simulink model "ParallelControl"  (R2015b)
settings: Solver=ode45  StartTime=0.0  StopTime=10  FixedStep=.002  RelTol=1e-3
settings Model: ExtModeTrigDuration=10000  Creator=smascaro  LastModifiedBy=Justin
settings SolverCC: PositivePriorityOrder=on
settings DataIOCC: LimitDataPoints=off  SaveFormat=Array  SignalLoggingSaveFormat=ModelDataLogs  SaveOutput=off  SaveTime=off
settings OptimizationCC: ExpressionDepthLimit=2147483647  InitFltsAndDblsToZero=on
settings DebuggingCC: SaveWithParameterizedLinksMsg=none  UnderspecifiedInitializationDetection=Classic  MergeDetectMultiDrivingBlocksExec=none  SignalResolutionControl=TryResolveAllWithWarning  SolverPrmCheckMsg=warning  MultiTaskDSMMsg=warning  MultiTaskCondExecSysMsg=none  FcnCallInpInsideContextMsg=UseLocalSettings  StateNameClashWarn=warning
settings HardwareCC: ProdBitPerPointer=32  ProdLargestAtomicFloat=None  ProdIntDivRoundTo=Undefined  ProdEndianess=Unspecified  ProdWordSize=32  ProdHWDeviceType=32-bit Generic  TargetBitPerPointer=64  TargetLongLongMode=on  TargetIntDivRoundTo=Zero  TargetEndianess=LittleEndian  TargetWordSize=64  TargetHWDeviceType=MATLAB Host
settings SFSimCC: SimParseCustomCode=off
settings RTWCC: SystemTargetFile=quarc_windows.tlc  TemplateMakefile=quarc_default_tmf  Description=QUARC Win32 Target
settings STFCustomTargetCC: TargetPreCompLibLocation=C:\PROGRA~3\QUARC\lib\2015b\windows\release  ConcurrentExecutionCompliant=off  SystemTargetFile=quarc_windows.tlc
settings GRTTargetCC: TargetPreCompLibLocation=C:\PROGRA~3\QUARC\lib\2015b\windows\release  ParMdlRefBuildCompliant=off  CompOptLevelCompliant=off  ConcurrentExecutionCompliant=off  GeneratePreprocessorConditionals=Disable all  CombineOutputUpdateFcns=off  MatFileLogging=off  GRTInterface=on  UseToolchainInfoCompliant=off  ExtMode=on  ExtModeMexFile=quarc_comm
settings ConfigComp: CovModelRefEnable=Off

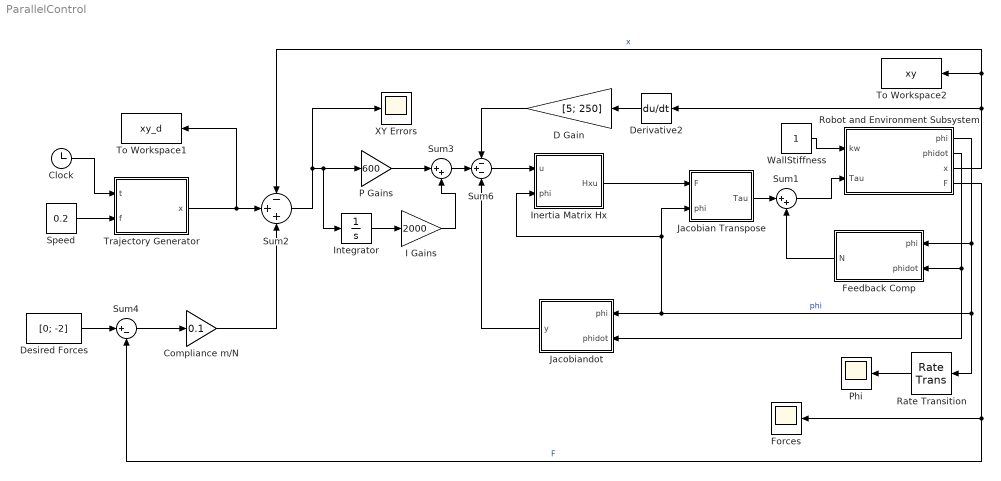
== system ParallelControl ==
  Clock : Clock
  "Compliance m/N " : Gain  Gain=0.1
  D Gain : Gain  Gain=[5; 250]
  Derivative2 : Derivative
  Desired Forces : Constant  Value=[0; -2]
  Feedback Comp : MATLAB Function  TreatAsAtomicUnit=on
  Forces : Scope
  I Gains : Gain  Gain=2000
  Inertia Matrix Hx : MATLAB Function  TreatAsAtomicUnit=on
  Integrator : Integrator
  Jacobian Transpose : MATLAB Function  TreatAsAtomicUnit=on
  Jacobiandot : MATLAB Function  TreatAsAtomicUnit=on
  P Gains : Gain  Gain=600
  Phi : Scope
      settings: AttributesFormatString=SampleTime =%<SampleTime>
  Rate Transition : RateTransition  OutPortSampleTimeOpt=Inherit  OutPortSampleTimeMultiple=10  OutPortSampleTime=0.05
  Robot and Environment Subsystem : Subsystem
  Speed : Constant  Value=0.2
      settings: AttributesFormatString=(circles/sec)
  Sum1 : Sum  Inputs=|++
  Sum2 : Sum  Inputs=-++
  Sum3 : Sum  Inputs=|++
  Sum4 : Sum  Inputs=|+-
  Sum6 : Sum  Inputs=-+-
  To Workspace1 : ToWorkspace  VariableName=xy_d  SampleTime=-1
  To Workspace2 : ToWorkspace  VariableName=xy  SampleTime=-1
  Trajectory Generator : MATLAB Function  TreatAsAtomicUnit=on
  WallStiffness : Constant
      settings: AttributesFormatString=(N/mm)
  XY Errors : Scope
  wires:
  Robot and Environment Subsystem/1(phi) -> Feedback Comp/1(phi), Jacobian Transpose/2(phi), Inertia Matrix Hx/2(phi), Jacobiandot/1(phi), Rate Transition/1  "phi"
  Robot and Environment Subsystem/3(x) -> To Workspace2/1, Sum2/1, Derivative2/1  "x"
  Clock/1 -> Trajectory Generator/1(t)
  Speed/1 -> Trajectory Generator/2(f)
  Rate Transition/1 -> Phi/1
  Robot and Environment Subsystem/4(F) -> Forces/1, Sum4/2  "F"
  Jacobian Transpose/1(Tau) -> Sum1/1
  Robot and Environment Subsystem/2(phidot) -> Jacobiandot/2(phidot), Feedback Comp/2(phidot)
  Feedback Comp/1(N) -> Sum1/2
  Sum1/1 -> Robot and Environment Subsystem/2(Tau)
  WallStiffness/1 -> Robot and Environment Subsystem/1(kw)
  Trajectory Generator/1(x) -> To Workspace1/1, Sum2/2
  Derivative2/1 -> D Gain/1
  Desired Forces/1 -> Sum4/1
  Sum4/1 -> "Compliance m/N "/1
  D Gain/1 -> Sum6/1
  Sum6/1 -> Inertia Matrix Hx/1(u)
  Inertia Matrix Hx/1(Hxu) -> Jacobian Transpose/1(F)
  "Compliance m/N "/1 -> Sum2/3
  Jacobiandot/1(y) -> Sum6/3
  Sum2/1 -> Integrator/1, P Gains/1, XY Errors/1
  Integrator/1 -> I Gains/1
  P Gains/1 -> Sum3/1
  Sum3/1 -> Sum6/2
  I Gains/1 -> Sum3/2

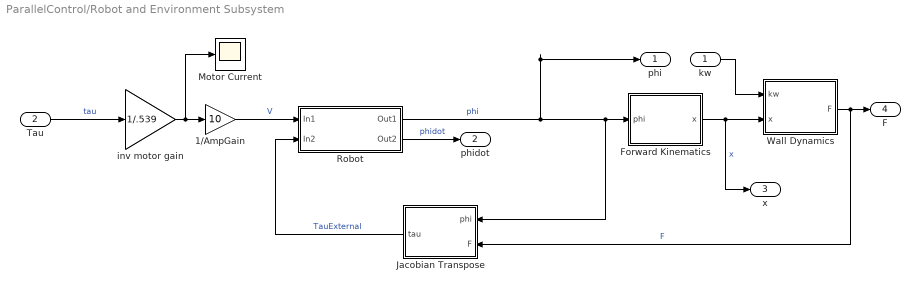
== system ParallelControl/Robot and Environment Subsystem ==
  kw : Inport
  Tau : Inport  Port=2
  1/AmpGain : Gain  Gain=10
  Forward Kinematics : MATLAB Function  TreatAsAtomicUnit=on
  Jacobian Transpose : MATLAB Function  TreatAsAtomicUnit=on
  Motor Current : Scope
  Robot : Subsystem
      mask Display: disp('Manipulator')
  Wall Dynamics : MATLAB Function  TreatAsAtomicUnit=on
  inv motor gain : Gain  Gain=1/.539
  phi : Outport
  phidot : Outport  Port=2
  x : Outport  Port=3
  F : Outport  Port=4
  wires:
  Robot/1(Out1) -> phi/1, Jacobian Transpose/1(phi), Forward Kinematics/1(phi)  "phi"
  Forward Kinematics/1(x) -> x/1, Wall Dynamics/2(x)  "x"
  Wall Dynamics/1(F) -> Jacobian Transpose/2(F), F/1  "F"
  inv motor gain/1 -> 1/AmpGain/1, Motor Current/1
  1/AmpGain/1 -> Robot/1(In1)  "V"
  kw/1 -> Wall Dynamics/1(kw)
  Robot/2(Out2) -> phidot/1  "phidot"
  Tau/1 -> inv motor gain/1  "tau"
  Jacobian Transpose/1(tau) -> Robot/2(In2)  "TauExternal"

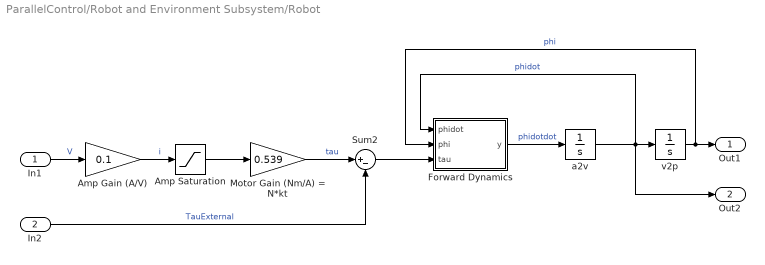
== system ParallelControl/Robot and Environment Subsystem/Robot ==
  In1 : Inport
  In2 : Inport  Port=2
  Amp Saturation : Saturate  UpperLimit=1  LowerLimit=-1  ZeroCross=off
  Amp Gain (A/V) : Gain  Gain=0.1
  Forward Dynamics : MATLAB Function  TreatAsAtomicUnit=on
  Motor Gain (Nm/A) = N*kt : Gain  Gain=0.539
  Sum2 : Sum  Inputs=|+-
  a2v : Integrator
  v2p : Integrator  InitialCondition=[0.3109;-0.4922]
  Out1 : Outport
  Out2 : Outport  Port=2
  wires:
  Forward Dynamics/1(y) -> a2v/1  "phidotdot"
  a2v/1 -> Out2/1, Forward Dynamics/1(phidot), v2p/1  "phidot"
  v2p/1 -> Out1/1, Forward Dynamics/2(phi)  "phi"
  In1/1 -> Amp Gain (A/V)/1  "V"
  Amp Saturation/1 -> Motor Gain (Nm/A) = N*kt/1
  Amp Gain (A/V)/1 -> Amp Saturation/1  "i"
  Sum2/1 -> Forward Dynamics/3(tau)
  Motor Gain (Nm/A) = N*kt/1 -> Sum2/1  "tau"
  In2/1 -> Sum2/2  "TauExternal"

== matlab function ParallelControl/Robot and Environment Subsystem/Jacobian Transpose ==
  settings: fimath=|
      | fimath(...
      | 'RoundMode', 'floor',...
      | 'OverflowMode', 'wrap',...
      | 'ProductMode', 'KeepLSB', 'ProductWordLength', 32,...
      | 'SumMode', 'KeepLSB', 'SumWordLength', 32,...
      | 'CastBeforeSum', false)
  data: tau output; phi input; F input
function tau = fcn(phi, F)
% This block supports an embeddable subset of the MATLAB language.
% See the help menu for details. 
a1=0.15;
a2=0.15;

J11 = -a1*sin(phi(1));
J12 = -a2*sin(phi(2));
J21 = a1*cos(phi(1));
J22 = a2*cos(phi(2));

J = [J11 J12; J21 J22];

tau = J'*F;

== matlab function ParallelControl/Robot and Environment Subsystem/Robot/Forward Dynamics ==
  settings: fimath=|
      | fimath(...
      | 'RoundMode', 'floor',...
      | 'OverflowMode', 'wrap',...
      | 'ProductMode', 'KeepLSB', 'ProductWordLength', 32,...
      | 'SumMode', 'KeepLSB', 'SumWordLength', 32,...
      | 'CastBeforeSum', false)
  data: phidot input double size=2; phi input double size=2; y output double size=2; tau input size=2
function y = fcn(phidot,phi,tau)
% This block supports an embeddable subset of the MATLAB language.
% See the help menu for details. 

a1 = 0.15;  % link 1 length
a2 = 0.15;  % link 2 length
m1 = 0.092;  % link 1 mass  
m2 = 0.077; % link 2 mas
r01 = 0.062; % link 1 center of mass
r12 = 0.036; % link 2 COM
I1 = 0.64e-3;  % link 1 inertia
I2 = 0.30e-3;  % link 2 inertia
Jm1 = 0.65e-6; % motor inertias
Jm2 = 0.65e-6;
b1 = 3.1e-6; % viscous damping constants
b2 = 3.1e-6;
c1 = 0.0001; % coulomb friction constants
c2 = 0.0001;
g = 9.8; % gravitational constant
N1 = 70; % gear ratios
N2 = 70;

H11 = N1^2*Jm1 + I1 + m2*a1^2;
H12 = a1*r12*m2*cos(phi(2)-phi(1));
H21 = H12;
H22 = N2^2*Jm2 + I2;
h = a1*r12*m2*sin(phi(2)-phi(1));
G1 = (r01*m1+a1*m2)*g*cos(phi(1));
G2 = r12*m2*g*cos(phi(2));
F1 = N1^2*b1*phidot(1) + N1*c1*sign(phidot(1));
F2 = N2^2*b2*phidot(2) + N2*c2*sign(phidot(2));

H = [H11 H12; H21 H22]; % inertia matrix
V = [0 -h ;h 0]*[phidot(1)^2;phidot(2)^2]; % centripetal torques
G = [G1;G2]; % gravity torques
F = [F1;F2]; % frictional torques

y = inv(H)*(tau - V - G - F); % y=phidotdot

== matlab function ParallelControl/Inertia Matrix Hx ==
  settings: fimath=|
      | fimath(...
      | 'RoundMode', 'floor',...
      | 'OverflowMode', 'wrap',...
      | 'ProductMode', 'KeepLSB', 'ProductWordLength', 32,...
      | 'SumMode', 'KeepLSB', 'SumWordLength', 32,...
      | 'CastBeforeSum', false)
  data: u input; phi input; Hxu output
function Hxu = fcn(u,phi)
% This block supports an embeddable subset of the MATLAB language.
% See the help menu for details. 


a1 = 0.15;  % link 1 length
a2 = 0.15;  % link 2 length
m1 = 0.092;  % link 1 mass  
m2 = 0.077; % link 2 mas
r01 = 0.062; % link 1 center of mass
r12 = 0.036; % link 2 COM
I1 = 0.64e-3;  % link 1 inertia
I2 = 0.30e-3;  % link 2 inertia
Jm1 = 0.65e-6; % motor inertias
Jm2 = 0.65e-6;

g = 9.8; % gravitational constant
N1 = 70; % gear ratios
N2 = 70;

H11 = N1^2*Jm1 + I1 + m2*a1^2;
H12 = a1*r12*m2*cos(phi(2)-phi(1));
H21 = H12;
H22 = N2^2*Jm2 + I2;

J11 = -a1*sin(phi(1));
J12 = -a2*sin(phi(2));
J21 = a1*cos(phi(1));
J22 = a2*cos(phi(2));

J = [J11 J12; J21 J22];  %Jacobian
H = [H11 H12; H21 H22];  %Inertia Matrix in Joint Space
Hx = inv(J')*H*inv(J);   %Inertia Matrix in Operational Space

Hxu = Hx*u;

== matlab function ParallelControl/Feedback Comp ==
  settings: fimath=|
      | fimath(...
      | 'RoundMode', 'floor',...
      | 'OverflowMode', 'wrap',...
      | 'ProductMode', 'KeepLSB', 'ProductWordLength', 32,...
      | 'SumMode', 'KeepLSB', 'SumWordLength', 32,...
      | 'CastBeforeSum', false)
  data: N output; phi input; phidot input
function N = fcn(phi, phidot)
% This block supports an embeddable subset of the MATLAB language.
% See the help menu for details. 


a1 = 0.15;  % link 1 length
a2 = 0.15;  % link 2 length
m1 = 0.092;  % link 1 mass  
m2 = 0.077; % link 2 mas
r01 = 0.062; % link 1 center of mass
r12 = 0.036; % link 2 COM
I1 = 0.64e-3;  % link 1 inertia
I2 = 0.30e-3;  % link 2 inertia
Jm1 = 0.65e-6; % motor inertias
Jm2 = 0.65e-6;
b1 = 3.1e-6; % viscous damping constants
b2 = 3.1e-6;
c1 = 0.0001; % coulomb friction constants
c2 = 0.0001;
g = 9.8; % gravitational constant
N1 = 70; % gear ratios
N2 = 70;

h = a1*r12*m2*sin(phi(2)-phi(1));
G1 = (r01*m1+a1*m2)*g*cos(phi(1));
G2 = r12*m2*g*cos(phi(2));
F1 = N1^2*b1*phidot(1) + N1*c1*sign(phidot(1));
F2 = N2^2*b2*phidot(2) + N2*c2*sign(phidot(2));

V = [0 -h ;h 0]*[phidot(1)^2;phidot(2)^2]; % centripetal torques
G = [G1;G2]; % gravity torques
F = [F1;F2]; % frictional torques

N = V + G + F;

== matlab function ParallelControl/Robot and Environment Subsystem/Wall Dynamics ==
  settings: fimath=|
      | fimath(...
      | 'RoundMode', 'floor',...
      | 'OverflowMode', 'wrap',...
      | 'ProductMode', 'KeepLSB', 'ProductWordLength', 32,...
      | 'SumMode', 'KeepLSB', 'SumWordLength', 32,...
      | 'CastBeforeSum', false)
  data: kw input; x input; F output
function F = fcn(kw,x)
% This block supports an embeddable subset of the MATLAB language.
% See the help menu for details. 

% kw = wall stiffness in N/mm, e.g. 1 N/mm

F = [0;0];
bw = 0;

if x(2)<-0.025
    F(2) = (kw*1000)*(x(2)+0.025);
end

== matlab function ParallelControl/Jacobian Transpose ==
  settings: fimath=|
      | fimath(...
      | 'RoundMode', 'floor',...
      | 'OverflowMode', 'wrap',...
      | 'ProductMode', 'KeepLSB', 'ProductWordLength', 32,...
      | 'SumMode', 'KeepLSB', 'SumWordLength', 32,...
      | 'CastBeforeSum', false)
  data: F input; Tau output; phi input
function Tau = fcn(F,phi)
% This block supports an embeddable subset of the MATLAB language.
% See the help menu for details. 
a1=0.15;
a2=0.15;

J11 = -a1*sin(phi(1));
J12 = -a2*sin(phi(2));
J21 = a1*cos(phi(1));
J22 = a2*cos(phi(2));

J = [J11 J12; J21 J22];

Tau = J'*F;

== matlab function ParallelControl/Trajectory Generator ==
  settings: fimath=|
      | fimath(...
      | 'RoundMode', 'floor',...
      | 'OverflowMode', 'wrap',...
      | 'ProductMode', 'KeepLSB', 'ProductWordLength', 32,...
      | 'SumMode', 'KeepLSB', 'SumWordLength', 32,...
      | 'CastBeforeSum', false)
  data: x output; t input; f input
function x = fcn(t,f)
% This block supports an embeddable subset of the MATLAB language.
% See the help menu for details. 
x = [0;0];

h = -0.025; % wall height

if t<0.5  % accelerate into circling trajectory
    x(1) = 0.075*cos(2*pi*f*t^2) + 0.2;
    x(2) = h;
else  % constant speed circling of-  radius 0.075 about x=[0.125,0.1]
    x(1) = 0.075*cos(2*pi*f*(t-0.25)) + 0.2;
    x(2) = h;
end

== matlab function ParallelControl/Jacobiandot ==
  settings: fimath=|
      | fimath(...
      | 'RoundMode', 'floor',...
      | 'OverflowMode', 'wrap',...
      | 'ProductMode', 'KeepLSB', 'ProductWordLength', 32,...
      | 'SumMode', 'KeepLSB', 'SumWordLength', 32,...
      | 'CastBeforeSum', false)
  data: y output; phi input; phidot input
function y = fcn(phi, phidot)
% This block supports an embeddable subset of the MATLAB language.
% See the help menu for details. 
a1=0.15;
a2=0.15;

% J11 = -a1*sin(phi(1));
% J12 = -a2*sin(phi(2));
% J21 = a1*cos(phi(1));
% J22 = a2*cos(phi(2));

Jdot11 = -a1*cos(phi(1))*phidot(1);
Jdot12 = -a2*cos(phi(2))*phidot(2);
Jdot21 = -a1*sin(phi(1))*phidot(1);
Jdot22 = -a1*sin(phi(2))*phidot(2);

Jdot = [Jdot11 Jdot12; Jdot21 Jdot22];

y = Jdot*phidot;

== matlab function ParallelControl/Robot and Environment Subsystem/Forward Kinematics ==
  settings: fimath=|
      | fimath(...
      | 'RoundMode', 'floor',...
      | 'OverflowMode', 'wrap',...
      | 'ProductMode', 'KeepLSB', 'ProductWordLength', 32,...
      | 'SumMode', 'KeepLSB', 'SumWordLength', 32,...
      | 'CastBeforeSum', false)
  data: x output; phi input
function x = fcn(phi)
% This block supports an embeddable subset of the MATLAB language.
% See the help menu for details. 

a1=0.15;
a2=0.15;
x = [0;0];
x(1) = a1*cos(phi(1))+a2*cos(phi(2));
x(2) = a1*sin(phi(1))+a2*sin(phi(2));
